simulink model "Reductor1"  (R2023a)
settings: Solver=VariableStepAuto  StartTime=0.0  StopTime=10.0  RelTol=1e-3
settings Model: Creator=mrrom  LastModifiedBy=mrrom

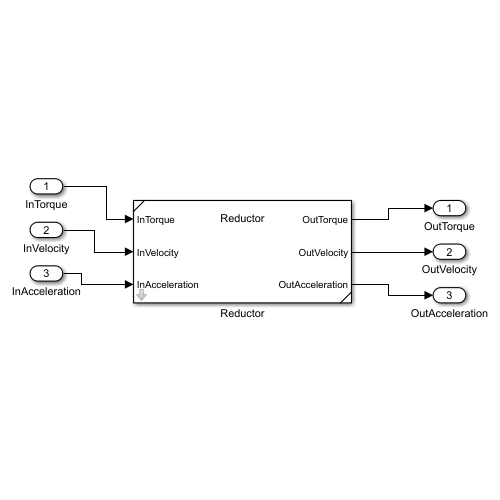
[thumbnail: Simulink's stored preview of the top-level diagram]
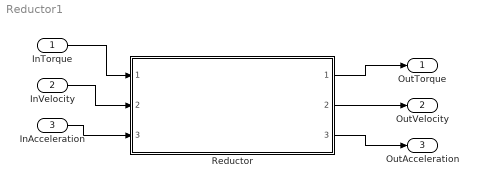
== system Reductor1 ==
  InTorque : Inport
  InVelocity : Inport  Port=2
  InAcceleration : Inport  Port=3
  Reductor : Subsystem  ReferencedSubsystem=Reductor  i_gear=100  J_gear=2.4e-6  vis_friction_coef_gear=3e-3
  OutTorque : Outport
  OutVelocity : Outport  Port=2
  OutAcceleration : Outport  Port=3
  wires:
  InTorque/1 -> Reductor/1
  InVelocity/1 -> Reductor/2
  InAcceleration/1 -> Reductor/3
  Reductor/1 -> OutTorque/1
  Reductor/2 -> OutVelocity/1
  Reductor/3 -> OutAcceleration/1
